simulink model "CompleteModelWindUp"  (R2019b)
settings: Solver=VariableStepAuto  StartTime=0.0  StopTime=1000  RelTol=1e-3
values from neighbouring files (symbols this model uses):
  A = [-0.322 0.052 0.028 -1.12 0.002;     0 0 1 -0.001 0;     -10.6 0 -2.87 0.46 -0.65;     6.87 0 -0.04 -0.32 -0.02;     0 0 0 0 -7.5]    [A2.m]    (also in model.m = [-0.322 0.052   0.028   -1.12   0.002; prob3sim.m)
  B = [0 0 0 0 7.5]'    [A2.m]    (also in model.m = [0; 0; 0; 0; 7.5]; prob3sim.m)
  C = [eye(4,5)]    [A2.m]    (also in model.m = cat(2, eye(4), zeros(4,1)); prob3sim.m)
  D = [0 0 0 0]'    [A2.m]    (also in prob3sim.m)
  k_dPhi = (2*z_rollDamp*omeg_NatRoll - a_phi1)/(a_phi2)    [A2.m]    (also in prob3sim.m)
  k_fPsi = 100000000000    [A2.m]    (also in prob3sim.m)
  k_iPhi = 0    [A2.m]    (also in prob3sim.m)
  k_iPsi = omeg_NatPsi^2*(V_g/g)    [A2.m]    (also in prob3sim.m)
  k_pPhi = (z_aMax/e_rollMax)*sign(a_phi2)    [A2.m]    (also in prob3sim.m)
  k_pPsi = 2*z_courseDamp*omeg_NatPsi*(V_g/g)    [A2.m]    (also in prob3sim.m)
libraries: simulink_extras x4
settings Model: Creator=Robert  LastModifiedBy=ola
settings DataIOCC: ReturnWorkspaceOutputs=off
settings DebuggingCC: UnderSpecifiedDimensionMsg=warning  ArithmeticOperatorsInVariantConditions=warning
settings SFSimCC: CustomCodeUndefinedFunction=UseInterfaceOnly

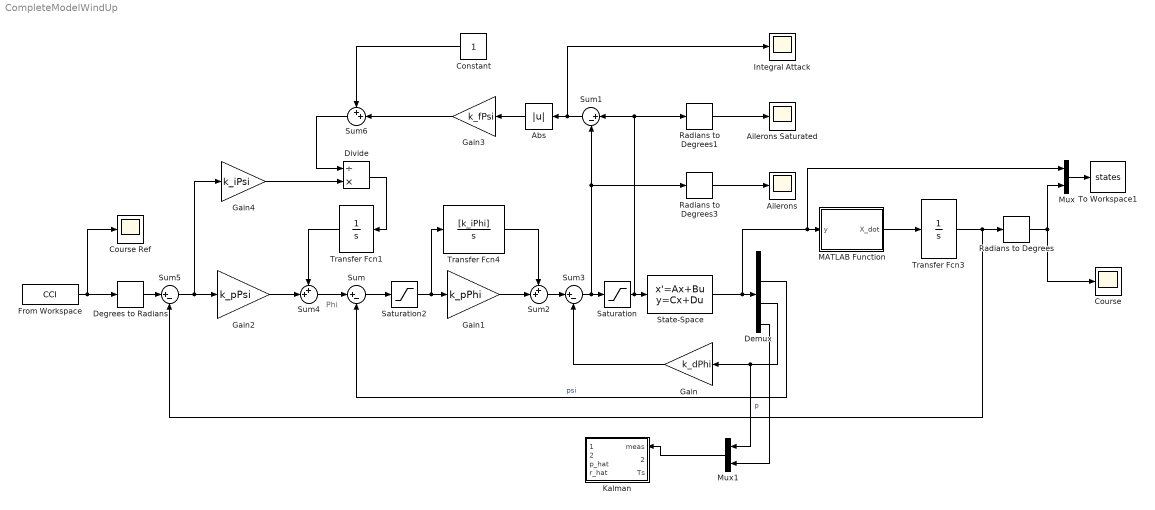
== system CompleteModelWindUp ==
  note: Phi
  Abs : Abs
  Ailerons : Scope
  "Ailerons Saturated " : Scope
  Constant : Constant
  "Course " : Scope
  "Course Ref " : Scope
  Degrees to Radians : simulink_extras/Transformations/Degrees to Radians
  Demux : Demux
  Divide : Product  Inputs=/*
  From Workspace : FromWorkspace  VariableName=CCI  SampleTime=0  Interpolate=off  OutputAfterFinalValue=Holding final value
  Gain : Gain  Gain=k_dPhi
  Gain1 : Gain  Gain=k_pPhi
  Gain2 : Gain  Gain=k_pPsi
  Gain3 : Gain  Gain=k_fPsi
  Gain4 : Gain  Gain=k_iPsi
  "Integral Attack " : Scope
  Kalman : MATLAB Function  TreatAsAtomicUnit=on
  MATLAB Function : MATLAB Function  TreatAsAtomicUnit=on
  Mux : Mux  Inputs=2
  Mux1 : Mux  Inputs=2
  Radians to Degrees : simulink_extras/Transformations/Radians to Degrees
  Radians to Degrees1 : simulink_extras/Transformations/Radians to Degrees
  Radians to Degrees3 : simulink_extras/Transformations/Radians to Degrees
  Saturation : Saturate  UpperLimit=30*(pi/180)  LowerLimit=-30*(pi/180)
  Saturation2 : Saturate  UpperLimit=15*(pi/180)  LowerLimit=-15*(pi/180)
  State-Space : StateSpace  A=A  B=B  C=C  D=D  InitialCondition=0
  Sum{,1,3,5} (4 alike) : Sum  Inputs=|+-
  Sum2 : Sum  Inputs=++|
  Sum4 : Sum  Inputs=++|
  Sum6 : Sum  Inputs=++|
  To Workspace1 : ToWorkspace  VariableName=states  SaveFormat=Timeseries  SampleTime=-1
  Transfer Fcn1 : TransferFcn  Denominator=[1,0]
  Transfer Fcn3 : TransferFcn  Denominator=[1,0]
  Transfer Fcn4 : TransferFcn  Numerator=[k_iPhi]  Denominator=[1 0]
  wires:
  Transfer Fcn3/1 -> Sum5/2, Radians to Degrees/1
  Sum/1 -> Saturation2/1
  Gain2/1 -> Sum4/2
  Transfer Fcn4/1 -> Sum2/1
  Sum4/1 -> Sum/1
  Gain1/1 -> Sum2/2
  Sum5/1 -> Gain4/1, Gain2/1
  State-Space/1 -> Mux/1, MATLAB Function/1(y), Demux/1
  Demux/2 -> Sum/2  "psi"
  Sum2/1 -> Sum3/1
  Gain/1 -> Sum3/2
  Demux/3 -> Mux1/1, Gain/1  "p"
  Sum3/1 -> Radians to Degrees3/1, Sum1/2, Saturation/1
  Saturation/1 -> Radians to Degrees1/1, Sum1/1, State-Space/1
  MATLAB Function/1(X_dot) -> Transfer Fcn3/1
  From Workspace/1 -> "Course Ref "/1, Degrees to Radians/1
  Degrees to Radians/1 -> Sum5/1
  Radians to Degrees/1 -> Mux/2, "Course "/1
  Sum1/1 -> Abs/1, "Integral Attack "/1
  Gain4/1 -> Divide/2
  Divide/1 -> Transfer Fcn1/1
  Transfer Fcn1/1 -> Sum4/1
  Radians to Degrees1/1 -> "Ailerons Saturated "/1
  Saturation2/1 -> Transfer Fcn4/1, Gain1/1
  Radians to Degrees3/1 -> Ailerons/1
  Abs/1 -> Gain3/1
  Constant/1 -> Sum6/1
  Gain3/1 -> Sum6/2
  Sum6/1 -> Divide/1
  Mux/1 -> To Workspace1/1
  Demux/4 -> Mux1/2
  Mux1/1 -> Kalman/1(meas)

== matlab function CompleteModelWindUp/Kalman ==
  data: meas input; beta_hat output; delta_a input; Ts input; phi_hat output; p_hat output; r_hat output


function [beta_hat, phi_hat, p_hat, r_hat] = Kalman(meas, delta_a, Ts)

    % initialize filter
    P_0 = zeros(4);
    x_0 = zeros(4,1);
    if Ts == 0
        P_bar = P_0;
        x_bar = x_0;
        P_hat = P_0;
        x_hat = x_0;
    end

    % covariance noise
    q = 1;
    r = 1;

    model = EKF(airplaneModel(q, r));
    
    [x_hat, P_hat] = model.update(meas, x_bar, P_bar);%... update
    NEES(k) = ((xhat(1:4,k)-xbar(1:4,k))')*inv(Pbar(1:4,1:4,k))*(xhat(1:4,k) - xbar(1:4,k));%... 
    NEESpos(k) = ((xhat(1:2,k)-xbar(1:2,k))')*inv(Pbar(1:2,1:2,k))*(xhat(1:2,k) - xbar(1:2,k));%...
    NEESvel(k) = ((xhat(3:4,k)-xbar(3:4,k))')*inv(Pbar(3:4,3:4,k))*(xhat(3:4,k) - xbar(3:4,k));%...
    if k < K
        [xbar(:, k+1), Pbar(:, :, k+1)] = tracker{s}.predict(xhat(:,k), Phat(:,:,k), Ts);%... predict
    end    
    

y = u;

== matlab function CompleteModelWindUp/MATLAB Function ==
  data: y input; X_dot output
function X_dot = fcn(y)
    g=9.81;
    V_g=580*(1/3.6);
X_dot = (g/V_g)*tan(y(2)+1.5*(pi/180))*cos(y(1));
